simulink model "DriveSystem"  (R2018b)
settings: Solver=FixedStepAuto  StartTime=0.0  StopTime=10.0  FixedStep=stepsize  RelTol=1e-3
undefined symbols (not defined in the file): d_visc, i_Getriebe, I_max_eff, J_gesamt, K_m, K_p, K_pi, K_s, k_stat, K_v, n_max, R, R_Trommel, T_el, T_i_control, T_n, T_ni, T_tot, T_v_control, T_x_control
libraries: simulink x3
settings Model: Creator=ac123748  LastModifiedBy=ac123748

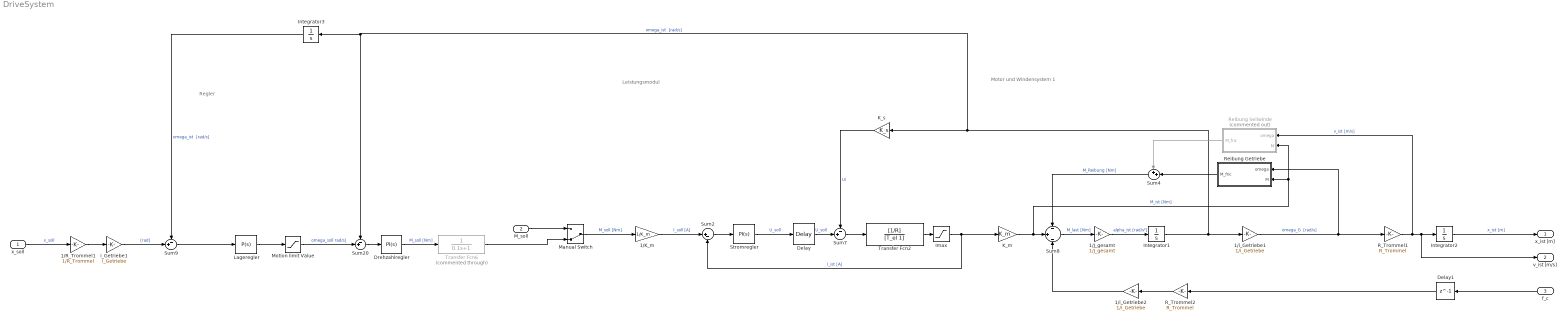
== system DriveSystem ==
  note: Motor und Windensystem 1
  note: Regler
  note: Leistungsmodul
  x_soll : Inport
  M_soll : Inport  Port=2
  f_c : Inport  Port=3
  1/J_gesamt : Gain  Gain=1/J_gesamt
  1/K_m : Gain  Gain=1/K_m
  1/R_Trommel1 : Gain  Gain=1/R_Trommel
  1/i_Getriebe1 : Gain  Gain=1/i_Getriebe
  1/i_Getriebe2 : Gain  Gain=1/i_Getriebe
  Delay : TransportDelay  DelayTime=T_tot
  Delay1 : Delay  DelayLength=1
  Drehzahlregler : simulink/Continuous/PID Controller  Controller=PI  Form=Ideal  TimeDomain=Continuous-time  SampleTime=T_v_control  IntegratorMethod=Forward Euler  FilterMethod=Forward Euler  ControllerParametersSource=internal  P=K_p  I=1/T_n  D=0  UseFilter=on  N=100  TunerSelectOption=Transfer Function Based (PID Tuner App)  InitialConditionSource=internal  InitialConditionForIntegrator=0  InitialConditionForFilter=0  DifferentiatorICPrevScaledInput=0  ExternalReset=none  TrackingMode=off  Kt=1  LimitOutput=off  UpperSaturationLimit=inf  LowerSaturationLimit=-inf  LinearizeAsGain=on  AntiWindupMode=none  Kb=1  POutMin=[]  POutMax=[]  IOutMin=[]  IOutMax=[]  DOutMin=[]  DOutMax=[]  NOutMin=[]  NOutMax=[]  SumOutMin=[]  SumOutMax=[]  SaturationOutMin=[]  SaturationOutMax=[]  PParamMin=[]  PParamMax=[]  IParamMin=[]  IParamMax=[]  DParamMin=[]  DParamMax=[]  NParamMin=[]  NParamMax=[]  KbParamMin=[]  KbParamMax=[]  KtParamMin=[]  KtParamMax=[]  KbOutMin=[]  KbOutMax=[]  KtOutMin=[]  KtOutMax=[]  IntegratorOutMin=[]  IntegratorOutMax=[]  FilterOutMin=[]  FilterOutMax=[]  SumI1OutMin=[]  SumI1OutMax=[]  SumI2OutMin=[]  SumI2OutMax=[]  SumI3OutMin=[]  SumI3OutMax=[]  SumI4OutMin=[]  SumI4OutMax=[]  SumDOutMin=[]  SumDOutMax=[]  DifferentiatorOutMin=[]  DifferentiatorOutMax=[]  FilterDiffOutCoefMin=[]  FilterDiffOutCoefMax=[]  ReciprocalOutMin=[]  ReciprocalOutMax=[]  SumDenOutMin=[]  SumDenOutMax=[]  SumNumOutMin=[]  SumNumOutMax=[]  DivideOutMin=[]  DivideOutMax=[]  IntegratorContinuousStateAttributes=''  IntegratorStateMustResolveToSignalObject=off  IntegratorRTWStateStorageClass=Auto  FilterContinuousStateAttributes=''  FilterStateMustResolveToSignalObject=off  FilterRTWStateStorageClass=Auto  ParallelPVariant=Passthrough  IdealPVariant=InternalParameters  IVariant=InternalParameters  DVariant=Disabled  IntegratorVariant=Continuous  SatVariant=Disabled  AWVariant=Passthrough  PCopyVariant=Disabled  TRVariant=Disabled  FdbkBlocksVariant=Forward  IdealPFdbkVariant=Disabled  SatFdbkVariant=Disabled  DerivativeFilterVariant=Disabled  NVariant=Disabled  NCopyVariant=Disabled_SignalSpec  FilterICVariant=Disabled  IntegratorICVariant=InternalICs  ExternalResetVariant=Disabled  TRSumVariant=Passthrough  SumFdbkVariant=Disabled  SumVariant=Sum_PI
  Imax : Saturate  UpperLimit=I_max_eff  LowerLimit=-I_max_eff
  Integrator1 : Integrator
  Integrator2 : Integrator
  Integrator3 : Integrator
  K_m : Gain  Gain=K_m
  K_s : Gain  Gain=K_s
  Lageregler : simulink/Continuous/PID Controller  Controller=P  Form=Ideal  TimeDomain=Continuous-time  SampleTime=T_x_control  IntegratorMethod=Forward Euler  FilterMethod=Forward Euler  ControllerParametersSource=internal  P=K_v  I=1  D=0  UseFilter=on  N=100  TunerSelectOption=Transfer Function Based (PID Tuner App)  InitialConditionSource=internal  InitialConditionForIntegrator=0  InitialConditionForFilter=0  DifferentiatorICPrevScaledInput=0  ExternalReset=none  TrackingMode=off  Kt=1  LimitOutput=off  UpperSaturationLimit=inf  LowerSaturationLimit=-inf  LinearizeAsGain=on  AntiWindupMode=none  Kb=1  POutMin=[]  POutMax=[]  IOutMin=[]  IOutMax=[]  DOutMin=[]  DOutMax=[]  NOutMin=[]  NOutMax=[]  SumOutMin=[]  SumOutMax=[]  SaturationOutMin=[]  SaturationOutMax=[]  PParamMin=[]  PParamMax=[]  IParamMin=[]  IParamMax=[]  DParamMin=[]  DParamMax=[]  NParamMin=[]  NParamMax=[]  KbParamMin=[]  KbParamMax=[]  KtParamMin=[]  KtParamMax=[]  KbOutMin=[]  KbOutMax=[]  KtOutMin=[]  KtOutMax=[]  IntegratorOutMin=[]  IntegratorOutMax=[]  FilterOutMin=[]  FilterOutMax=[]  SumI1OutMin=[]  SumI1OutMax=[]  SumI2OutMin=[]  SumI2OutMax=[]  SumI3OutMin=[]  SumI3OutMax=[]  SumI4OutMin=[]  SumI4OutMax=[]  SumDOutMin=[]  SumDOutMax=[]  DifferentiatorOutMin=[]  DifferentiatorOutMax=[]  FilterDiffOutCoefMin=[]  FilterDiffOutCoefMax=[]  ReciprocalOutMin=[]  ReciprocalOutMax=[]  SumDenOutMin=[]  SumDenOutMax=[]  SumNumOutMin=[]  SumNumOutMax=[]  DivideOutMin=[]  DivideOutMax=[]  IntegratorContinuousStateAttributes=''  IntegratorStateMustResolveToSignalObject=off  IntegratorRTWStateStorageClass=Auto  FilterContinuousStateAttributes=''  FilterStateMustResolveToSignalObject=off  FilterRTWStateStorageClass=Auto  ParallelPVariant=InternalParameters  IdealPVariant=Disabled  IVariant=Disabled  DVariant=Disabled  IntegratorVariant=Disabled  SatVariant=Disabled  AWVariant=Disabled  PCopyVariant=Disabled  TRVariant=Disabled  FdbkBlocksVariant=Forward  IdealPFdbkVariant=Disabled  SatFdbkVariant=Disabled  DerivativeFilterVariant=Disabled  NVariant=Disabled  NCopyVariant=Disabled_SignalSpec  FilterICVariant=Disabled  IntegratorICVariant=Disabled  ExternalResetVariant=Disabled  TRSumVariant=Passthrough  SumFdbkVariant=Disabled  SumVariant=Passthrough_P
  Manual Switch : ManualSwitch  CurrentSetting=0
  Motion limit Value : Saturate  UpperLimit=n_max  LowerLimit=-n_max
  R_Trommel1 : Gain  Gain=R_Trommel
  R_Trommel2 : Gain  Gain=R_Trommel
  Reibung Getriebe : Subsystem
  Reibung Seilwinde : Subsystem  Commented=on
  Stromregler : simulink/Continuous/PID Controller  Controller=PI  Form=Ideal  TimeDomain=Continuous-time  SampleTime=T_i_control  IntegratorMethod=Forward Euler  FilterMethod=Forward Euler  ControllerParametersSource=internal  P=K_pi  I=1/T_ni  D=0  UseFilter=on  N=100  TunerSelectOption=Transfer Function Based (PID Tuner App)  InitialConditionSource=internal  InitialConditionForIntegrator=0  InitialConditionForFilter=0  DifferentiatorICPrevScaledInput=0  ExternalReset=none  TrackingMode=off  Kt=1  LimitOutput=off  UpperSaturationLimit=inf  LowerSaturationLimit=-inf  LinearizeAsGain=on  AntiWindupMode=none  Kb=1  POutMin=[]  POutMax=[]  IOutMin=[]  IOutMax=[]  DOutMin=[]  DOutMax=[]  NOutMin=[]  NOutMax=[]  SumOutMin=[]  SumOutMax=[]  SaturationOutMin=[]  SaturationOutMax=[]  PParamMin=[]  PParamMax=[]  IParamMin=[]  IParamMax=[]  DParamMin=[]  DParamMax=[]  NParamMin=[]  NParamMax=[]  KbParamMin=[]  KbParamMax=[]  KtParamMin=[]  KtParamMax=[]  KbOutMin=[]  KbOutMax=[]  KtOutMin=[]  KtOutMax=[]  IntegratorOutMin=[]  IntegratorOutMax=[]  FilterOutMin=[]  FilterOutMax=[]  SumI1OutMin=[]  SumI1OutMax=[]  SumI2OutMin=[]  SumI2OutMax=[]  SumI3OutMin=[]  SumI3OutMax=[]  SumI4OutMin=[]  SumI4OutMax=[]  SumDOutMin=[]  SumDOutMax=[]  DifferentiatorOutMin=[]  DifferentiatorOutMax=[]  FilterDiffOutCoefMin=[]  FilterDiffOutCoefMax=[]  ReciprocalOutMin=[]  ReciprocalOutMax=[]  SumDenOutMin=[]  SumDenOutMax=[]  SumNumOutMin=[]  SumNumOutMax=[]  DivideOutMin=[]  DivideOutMax=[]  IntegratorContinuousStateAttributes=''  IntegratorStateMustResolveToSignalObject=off  IntegratorRTWStateStorageClass=Auto  FilterContinuousStateAttributes=''  FilterStateMustResolveToSignalObject=off  FilterRTWStateStorageClass=Auto  ParallelPVariant=Passthrough  IdealPVariant=InternalParameters  IVariant=InternalParameters  DVariant=Disabled  IntegratorVariant=Continuous  SatVariant=Disabled  AWVariant=Passthrough  PCopyVariant=Disabled  TRVariant=Disabled  FdbkBlocksVariant=Forward  IdealPFdbkVariant=Disabled  SatFdbkVariant=Disabled  DerivativeFilterVariant=Disabled  NVariant=Disabled  NCopyVariant=Disabled_SignalSpec  FilterICVariant=Disabled  IntegratorICVariant=InternalICs  ExternalResetVariant=Disabled  TRSumVariant=Passthrough  SumFdbkVariant=Disabled  SumVariant=Sum_PI
  Sum2 : Sum  Inputs=|+-
  Sum20 : Sum  Inputs=-+|
  Sum4 : Sum  Inputs=++|
  Sum7 : Sum  Inputs=-+|
  Sum8 : Sum  Inputs=-|+|-
  Sum9 : Sum  Inputs=-+|
  Transfer Fcn2 : TransferFcn  Numerator=[1/R]  Denominator=[T_el 1]  ContinuousStateAttributes='current'
  Transfer Fcn6 : TransferFcn  Commented=through  Denominator=[0.1 1]
  i_Getriebe1 : Gain  Gain=i_Getriebe
  x_ist [m] : Outport
  v_ist [m/s] : Outport  Port=2
  wires:
  Drehzahlregler/1 -> Transfer Fcn6/1  "M_soll [Nm]"
  R_Trommel1/1 -> Reibung Seilwinde/1(omega), v_ist [m/s]/1, Integrator2/1  "v_ist [m/s]"
  i_Getriebe1/1 -> Sum9/2  "[rad]"
  1/i_Getriebe2/1 -> Sum8/3
  K_m/1 -> Reibung Getriebe/2(M), Reibung Seilwinde/2(M), Sum8/2  "M_ist [Nm]"
  Integrator1/1 -> 1/i_Getriebe1/1, Sum20/1, Integrator3/1, K_s/1  "omega_ist  [rad/s]"
  Transfer Fcn6/1 -> Manual Switch/2
  1/K_m/1 -> Sum2/1  "I_soll [A]"
  Integrator2/1 -> x_ist [m]/1  "x_ist [m]"
  1/J_gesamt/1 -> Integrator1/1  "alpha_ist [rad/s²]"
  Sum9/1 -> Lageregler/1
  Manual Switch/1 -> 1/K_m/1  "M_soll [Nm]"
  Sum7/1 -> Transfer Fcn2/1
  Sum8/1 -> 1/J_gesamt/1  "M_last [Nm]"
  Integrator3/1 -> Sum9/1  "omega_ist  [rad/s]"
  1/R_Trommel1/1 -> i_Getriebe1/1
  K_s/1 -> Sum7/1  "Ui"
  Imax/1 -> Sum2/2, K_m/1  "I_ist [A]"
  Reibung Seilwinde/1(M_fric) -> Sum4/1
  Delay/1 -> Sum7/2  "U_soll"
  x_soll/1 -> 1/R_Trommel1/1  "x_soll"
  Reibung Getriebe/1(M_fric) -> Sum4/2
  Lageregler/1 -> Motion limit Value/1
  Stromregler/1 -> Delay/1  "U_soll"
  Sum20/1 -> Drehzahlregler/1
  Sum2/1 -> Stromregler/1
  1/i_Getriebe1/1 -> R_Trommel1/1, Reibung Getriebe/1(omega)  "omega_G  [rad/s]"
  Sum4/1 -> Sum8/1  "M_Reibung [Nm]"
  R_Trommel2/1 -> 1/i_Getriebe2/1
  Transfer Fcn2/1 -> Imax/1
  Motion limit Value/1 -> Sum20/2  "omega_soll rad/s]"
  M_soll/1 -> Manual Switch/1
  f_c/1 -> Delay1/1
  Delay1/1 -> R_Trommel2/1

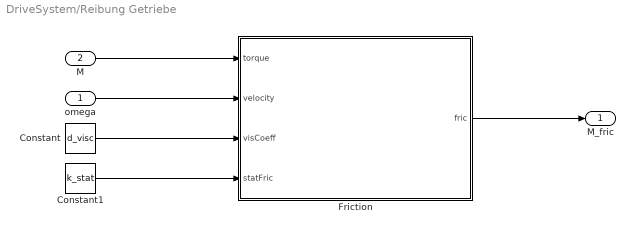
== system DriveSystem/Reibung Getriebe ==
  omega : Inport
  M : Inport  Port=2
  Constant : Constant  Value=d_visc
  Constant1 : Constant  Value=k_stat
  Friction : MATLAB Function  TreatAsAtomicUnit=on
  M_fric : Outport
  wires:
  Constant/1 -> Friction/3(visCoeff)
  Friction/1(fric) -> M_fric/1
  Constant1/1 -> Friction/4(statFric)
  omega/1 -> Friction/2(velocity)
  M/1 -> Friction/1(torque)

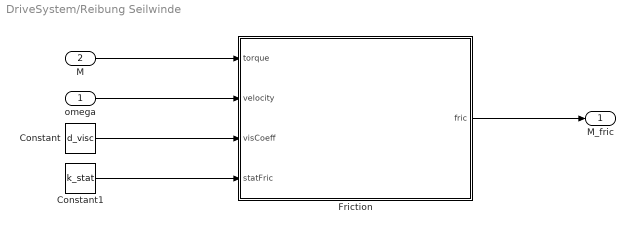
== system DriveSystem/Reibung Seilwinde ==
  omega : Inport
  M : Inport  Port=2
  Constant : Constant  Value=d_visc
  Constant1 : Constant  Value=k_stat
  Friction : MATLAB Function  TreatAsAtomicUnit=on
  M_fric : Outport
  wires:
  Constant/1 -> Friction/3(visCoeff)
  Friction/1(fric) -> M_fric/1
  Constant1/1 -> Friction/4(statFric)
  omega/1 -> Friction/2(velocity)
  M/1 -> Friction/1(torque)

== matlab function DriveSystem/Reibung Getriebe/Friction ==
  data: torque input; velocity input; visCoeff input; statFric input; fric output
function fric   = fcn(torque, velocity,visCoeff,statFric)

%   fc = 0.8*statFric;
  
  if abs(velocity) < 0.001
    if torque > statFric
      fric = statFric;
    elseif torque < -statFric
      fric = -statFric;
    else %-statFric < torque_R && torque_R < statFric
      fric = torque;
    end
    
  else %wheel_velocity_R > 0.1
%     fricR = (fc + (statFric-fc)*exp(-0.1*abs(wheel_velocity_R))) ...
%       *sign(wheel_velocity_R) + visCoeff*wheel_velocity_R;
    fric = statFric*sign(velocity) + visCoeff*velocity;
    
  end

end

== matlab function DriveSystem/Reibung Seilwinde/Friction ==
  data: torque input; velocity input; visCoeff input; statFric input; fric output
function fric   = fcn(torque, velocity,visCoeff,statFric)

%   fc = 0.8*statFric;
  
  if abs(velocity) < 0.001
    if torque > statFric
      fric = statFric;
    elseif torque < -statFric
      fric = -statFric;
    else %-statFric < torque_R && torque_R < statFric
      fric = torque;
    end
    
  else %wheel_velocity_R > 0.1
%     fricR = (fc + (statFric-fc)*exp(-0.1*abs(wheel_velocity_R))) ...
%       *sign(wheel_velocity_R) + visCoeff*wheel_velocity_R;
    fric = statFric*sign(velocity) + visCoeff*velocity;
    
  end

end
